simulink model "A02_L4"  (R2014b)
settings: Solver=ode113  StartTime=0.0  StopTime=4  MaxStep=0.01  RelTol=1e-5
values from neighbouring files (symbols this model uses):
  Feo = 5+3*a+b    (= 10)    [A03_L4_script.m]
  kp = 35-0.5*b    (= 32.5)    [A03_L4_script.m]
  kr = 10^3+2*a    (= 1000)    [A03_L4_script.m]
  m = 10+0.2*a+0.45*b    (= 12.25)    [A03_L4_script.m]
  v0 = 0    [A03_L4_script.m]
  x0 = 0    [A03_L4_script.m]
settings Model: Creator=User  LastModifiedBy=User

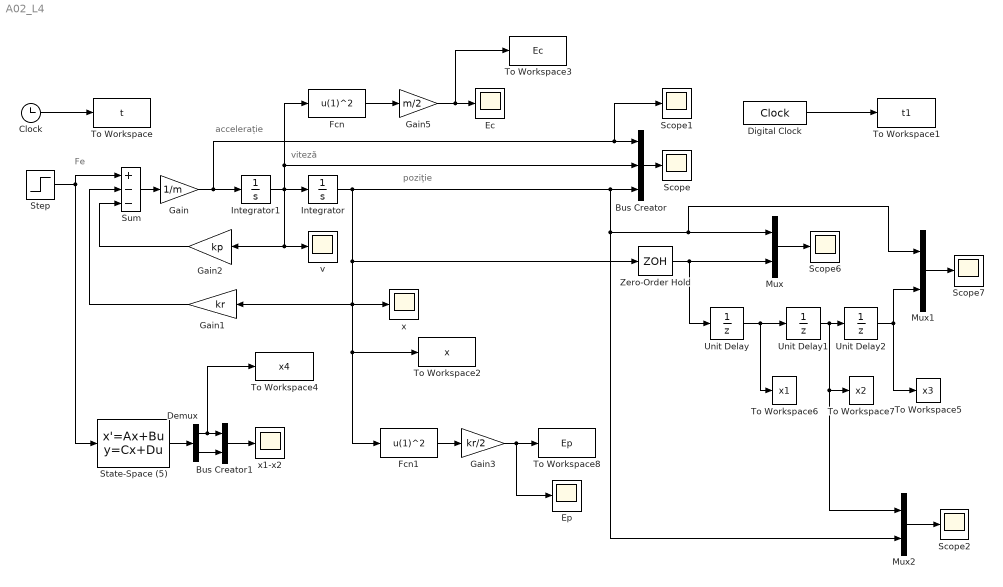
== system A02_L4 ==
  note: Fe
  note: poziție
  note: viteză
  note: accelerație
  Bus Creator : BusCreator  Inputs=3
  Bus Creator1 : BusCreator  Inputs=2
  Clock : Clock
  Demux : Demux  Outputs=2
  Digital Clock : DigitalClock  SampleTime=0.33
  Ec : Scope
      settings: SaveName=ScopeData4  MaxDataPoints=50000
  Ep : Scope
      settings: SaveName=ScopeData8  MaxDataPoints=50000
  Fcn : Fcn  Expr=u(1)^2
  Fcn1 : Fcn  Expr=u(1)^2
  Gain : Gain  Gain=1/m
  Gain1 : Gain  Gain=kr
  Gain2 : Gain  Gain=kp
  Gain3 : Gain  Gain=kr/2
  Gain5 : Gain  Gain=m/2
  Integrator : Integrator  InitialCondition=x0
  Integrator1 : Integrator  InitialCondition=v0
  Mux : Mux  Inputs=2
  Mux1 : Mux  Inputs=2
  Mux2 : Mux  Inputs=2
  Scope{,1..2,6..7} (5 alike) : Scope
      Scope2 settings: SaveName=ScopeData10  MaxDataPoints=50000
      Scope6 settings: SaveName=ScopeData6  MaxDataPoints=50000
      Scope7 settings: SaveName=ScopeData7  MaxDataPoints=50000
  State-Space (5) : StateSpace  A=[0 1;-kr/m -kp/m]  B=[0; 1/m]  C=[1 0; 0 1]  D=[0; 0]  X0=[x0; v0]
  Step : Step  After=Feo  SampleTime=0
  Sum : Sum  Inputs=|+--
  To Workspace : ToWorkspace  VariableName=t  SampleTime=-1
  To Workspace1 : ToWorkspace  VariableName=t1  SampleTime=-1
  To Workspace2 : ToWorkspace  VariableName=x  SampleTime=-1
  To Workspace3 : ToWorkspace  VariableName=Ec  SampleTime=-1
  To Workspace4 : ToWorkspace  VariableName=x4  SampleTime=-1
  To Workspace5 : ToWorkspace  VariableName=x3  SampleTime=-1
  To Workspace6 : ToWorkspace  VariableName=x1  SampleTime=-1
  To Workspace7 : ToWorkspace  VariableName=x2  SampleTime=-1
  To Workspace8 : ToWorkspace  VariableName=Ep  SampleTime=-1
  Unit Delay : UnitDelay  SampleTime=0.33
  Unit Delay1 : UnitDelay  SampleTime=0.33
  Unit Delay2 : UnitDelay  InitialCondition=0.02  SampleTime=0.33
  Zero-Order Hold : ZeroOrderHold  SampleTime=0.33
  v : Scope
      settings: SaveName=ScopeData2  MaxDataPoints=50000
  x : Scope
      settings: SaveName=ScopeData3  MaxDataPoints=50000
  x1-x2 : Scope
      settings: TickLabels=on  ShowLegends=on  SaveName=ScopeData5  MaxDataPoints=50000
  wires:
  Integrator1/1 -> Integrator/1, v/1, Gain2/1, Fcn/1, Bus Creator/2
  Sum/1 -> Gain/1
  Bus Creator/1 -> Scope/1
  Gain2/1 -> Sum/3
  Gain1/1 -> Sum/2
  Integrator/1 -> Zero-Order Hold/1, x/1, Fcn1/1, To Workspace2/1, Gain1/1, Mux2/2, Mux1/1, Mux/1, Bus Creator/3
  Gain/1 -> Scope1/1, Bus Creator/1, Integrator1/1
  Step/1 -> State-Space (5)/1, Sum/1
  Clock/1 -> To Workspace/1
  State-Space (5)/1 -> Demux/1
  Demux/1 -> To Workspace4/1, Bus Creator1/1
  Demux/2 -> Bus Creator1/2
  Bus Creator1/1 -> x1-x2/1
  Digital Clock/1 -> To Workspace1/1
  Zero-Order Hold/1 -> Mux/2, Unit Delay/1
  Mux/1 -> Scope6/1
  Unit Delay/1 -> To Workspace6/1, Unit Delay1/1
  Unit Delay1/1 -> Mux2/1, To Workspace7/1, Unit Delay2/1
  Unit Delay2/1 -> To Workspace5/1, Mux1/2
  Mux1/1 -> Scope7/1
  Fcn/1 -> Gain5/1
  Gain5/1 -> To Workspace3/1, Ec/1
  Fcn1/1 -> Gain3/1
  Gain3/1 -> Ep/1, To Workspace8/1
  Mux2/1 -> Scope2/1
